simulink model "metron"  (R2019b)
settings: Solver=VariableStepAuto  StartTime=0.0  StopTime=15  RelTol=1e-3
values from neighbouring files (symbols this model uses):
  c = set_controller()    [lab3.m]    (also in metronomo.m; set_controller.m = struct('name', 'Controlador'))
  s = rmfield(s, 'm')    [getWnfromSimulation.m]    (also in get_m_fromSimulation.m; lab3.m = set_system9(l_ls(2),m); lgetNLS.m = set_system9(new_l(j,i),s.m); metronomo.m = set_system9(l_nls(2),m))
undefined symbols (not defined in the file or in its folder): sgn
libraries: simulink x1
settings Model: Creator=joaotiagoalmeida  LastModifiedBy=joaotiagoalmeida

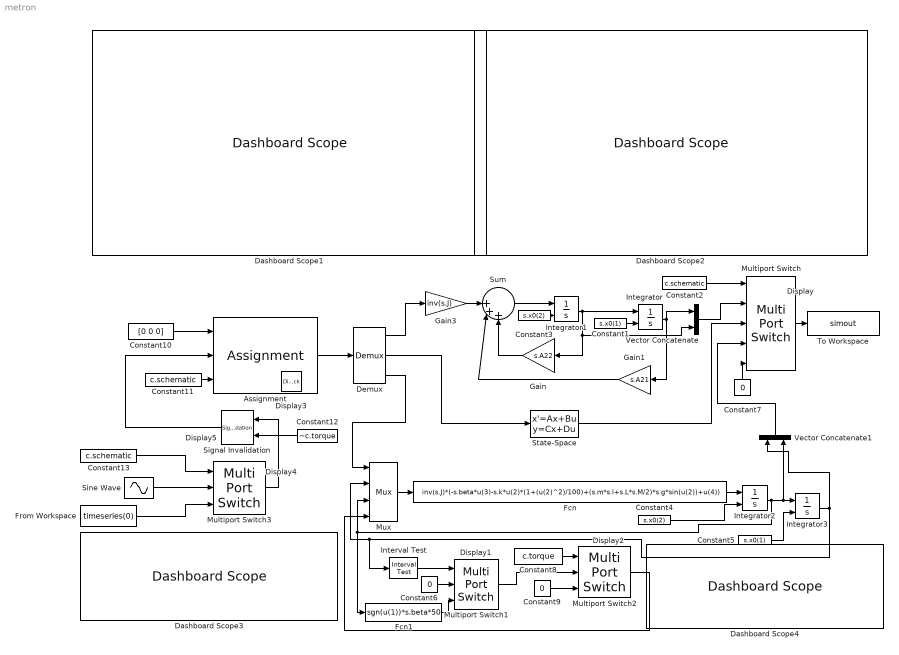
== system metron ==
  Assignment : Assignment  DiagnosticForDimensions=Warning  IndexOptions=Index vector (port)  Indices=[5 6 10]  OutputSizes=1
  Constant1 : Constant  Value=s.x0(1)  SampleTime=c.samptime
  Constant10 : Constant  Value=[0 0 0]  SampleTime=c.samptime
  Constant11 : Constant  Value=c.schematic  SampleTime=c.samptime
  Constant12 : Constant  Value=~c.torque  OutDataTypeStr=boolean  SampleTime=c.samptime
  Constant13 : Constant  Value=c.schematic  SampleTime=c.samptime
  Constant2 : Constant  Value=c.schematic  SampleTime=c.samptime
  Constant3 : Constant  Value=s.x0(2)  SampleTime=c.samptime
  Constant4 : Constant  Value=s.x0(2)  SampleTime=c.samptime
  Constant5 : Constant  Value=s.x0(1)  SampleTime=c.samptime
  Constant6 : Constant  Value=0  SampleTime=c.samptime
  Constant7 : Constant  Value=0  SampleTime=c.samptime
  Constant8 : Constant  Value=c.torque  SampleTime=c.samptime
  Constant9 : Constant  Value=0  SampleTime=c.samptime
  Dashboard Scope{1..4} (4 alike) : DashboardScope
  Demux : Demux  Outputs=3
  Display{,1..5} (6 alike) : DisplayBlock  LabelPosition=Hide  Format=short  Transparency=1
  Fcn : Fcn  Expr=inv(s.J)*(-s.beta*u(3)-s.k*u(2)*(1+(u(2)^2)/100)+(s.m*s.l+s.L*s.M/2)*s.g*sin(u(2))+u(4))
  Fcn1 : Fcn  Expr=sgn(u(1))*s.beta*50
  From Workspace : FromWorkspace  VariableName=timeseries(0)  SampleTime=c.samptime  OutputAfterFinalValue=Holding final value
  Gain : Gain  Gain=s.A22
  Gain1 : Gain  Gain=s.A21
  Gain3 : Gain  Gain=inv(s.J)
  Integrator : Integrator  InitialConditionSource=external
  Integrator1 : Integrator  InitialConditionSource=external  IgnoreLimit=on  ZeroCross=off
  Integrator2 : Integrator  InitialConditionSource=external  IgnoreLimit=on  ZeroCross=off
  Integrator3 : Integrator  InitialConditionSource=external
  Interval Test : simulink/Logic and Bit Operations/Interval Test  IntervalClosedRight=on  uplimit=c.torquelimit  IntervalClosedLeft=on  lowlimit=-c.torquelimit  OutDataTypeStr=boolean
  Multiport Switch : MultiPortSwitch  DataPortOrder=Specify indices  DataPortForDefault=Additional data port  DiagnosticForDefault=None
  Multiport Switch1 : MultiPortSwitch  DataPortOrder=Specify indices  DataPortIndices={0,1}  DiagnosticForDefault=None
  Multiport Switch2 : MultiPortSwitch  DataPortOrder=Specify indices  DataPortIndices={1,0}  DiagnosticForDefault=None
  Multiport Switch3 : MultiPortSwitch  DataPortOrder=Specify indices  DataPortIndices={[2],[1,3,4]}  DiagnosticForDefault=None  OutDataTypeStr=double
  Mux : Mux
  Signal Invalidation : SignalInvalidation  InvalidationPolicy=Replace
  Sine Wave : Sin  Frequency=pi*2  Samples=200  SampleTime=c.samptime
  State-Space : StateSpace  A=s.sys.A  B=s.sys.B  C=s.sys.C  D=s.sys.D  InitialCondition=s.x0
  Sum : Sum  Inputs=||+++
  To Workspace : ToWorkspace  VariableName=simout  SaveFormat=Timeseries  SampleTime=c.samptime
  Vector Concatenate : Concatenate
  Vector Concatenate1 : Concatenate
  wires:
  Gain3/1 -> Sum/1
  Sum/1 -> Integrator1/1
  Integrator1/1 -> Integrator/1, Vector Concatenate/2, Gain/1
  Multiport Switch/1 -> To Workspace/1
  Integrator/1 -> Vector Concatenate/1, Gain1/1
  Gain/1 -> Sum/3
  Gain1/1 -> Sum/2
  State-Space/1 -> Multiport Switch/3
  Constant2/1 -> Multiport Switch/1
  Constant1/1 -> Integrator/2
  Vector Concatenate/1 -> Multiport Switch/2
  Constant3/1 -> Integrator1/2
  Mux/1 -> Fcn/1
  Fcn/1 -> Integrator2/1
  Integrator2/1 -> Vector Concatenate1/2, Integrator3/1, Fcn1/1, Mux/3
  Constant4/1 -> Integrator2/2
  Constant5/1 -> Integrator3/2
  Integrator3/1 -> Mux/2, Interval Test/1, Vector Concatenate1/1
  Vector Concatenate1/1 -> Multiport Switch/4
  Interval Test/1 -> Multiport Switch1/1
  Constant7/1 -> Multiport Switch/5
  Constant6/1 -> Multiport Switch1/2
  Fcn1/1 -> Multiport Switch1/3
  Constant8/1 -> Multiport Switch2/1
  Multiport Switch1/1 -> Multiport Switch2/2
  Constant9/1 -> Multiport Switch2/3
  Multiport Switch2/1 -> Mux/4
  Assignment/1 -> Demux/1
  Constant10/1 -> Assignment/1
  Constant11/1 -> Assignment/3
  Demux/1 -> Gain3/1
  Demux/3 -> Mux/1
  Sine Wave/1 -> Multiport Switch3/2
  From Workspace/1 -> Multiport Switch3/3
  Demux/2 -> State-Space/1
  Constant12/1 -> Signal Invalidation/2
  Constant13/1 -> Multiport Switch3/1
  Multiport Switch3/1 -> Signal Invalidation/1
  Signal Invalidation/1 -> Assignment/2
